simulink model "test"  (R2018b)
settings: Solver=VariableStepAuto  StartTime=0.0  StopTime=10.0  RelTol=1e-3
libraries: S_TaLiRo x1
settings Model: Creator=claudio.menghi  LastModifiedBy=claudio.menghi

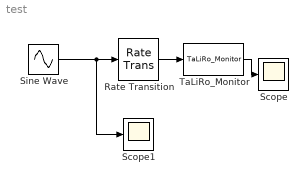
== system test ==
  Rate Transition : RateTransition
  Scope : Scope
  Scope1 : Scope
  Sine Wave : Sin  SampleTime=0
  TaLiRo_Monitor : S_TaLiRo/TaLiRo_Monitor  SFunctionModules=''
      settings: SourceProductName=S-TaLiRo
  wires:
  Sine Wave/1 -> Scope1/1, Rate Transition/1
  TaLiRo_Monitor/1 -> Scope/1
  Rate Transition/1 -> TaLiRo_Monitor/1
